simulink model "Pouziti_Discrete"  (R2020b)
settings: Solver=VariableStepAuto  StartTime=0.0  StopTime=10.0  RelTol=1e-3  EnableMultiTasking=on
PreLoadFcn:
  | T = 1;
  | Ts = 0.1;
CloseFcn:
  | clear T Ts
settings Model: Creator=Jirkovsk  LastModifiedBy=jirkovsky
settings DataIOCC: SaveTime=off  ReturnWorkspaceOutputs=off
settings OptimizationCC: LifeSpan=inf
settings DebuggingCC: SFUnexpectedBacktrackingDiag=warning  SFNoUnconditionalDefaultTransitionDiag=warning  SFExecutionAtInitializationDiag=none  ArithmeticOperatorsInVariantConditions=warning
settings SFSimCC: SimUseLocalCustomCode=off  CustomCodeUndefinedFunction=UseInterfaceOnly
settings RTWCC: RTWUseLocalCustomCode=off
settings CodeAppCC: StateflowObjectComments=on
settings GRTTargetCC: TargetLangStandard=C89/C90 (ANSI)
settings ConfigComp: CovMetricSettings=dw  CovSaveCumulativeToWorkspaceVar=on  CovSaveSingleToWorkspaceVar=on  CovExternalEMLEnable=off

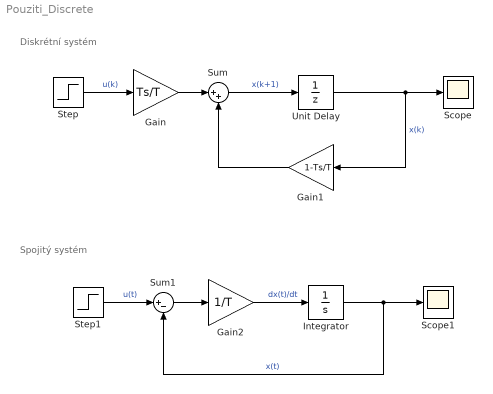
== system Pouziti_Discrete ==
  note: Diskrétní systém
  note: Spojitý systém
  Gain : Gain  Gain=Ts/T
  Gain1 : Gain  Gain=1-Ts/T
  Gain2 : Gain  Gain=1/T
  Integrator : Integrator
  Scope : Scope
  Scope1 : Scope
  Step : Step  SampleTime=Ts
  Step1 : Step  SampleTime=0
  Sum : Sum  Inputs=|++
  Sum1 : Sum  Inputs=|+-
  Unit Delay : UnitDelay  SampleTime=Ts  HasFrameUpgradeWarning=on
  wires:
  Step/1 -> Gain/1  "u(k)"
  Gain/1 -> Sum/1
  Sum/1 -> Unit Delay/1  "x(k+1)"
  Gain1/1 -> Sum/2
  Gain2/1 -> Integrator/1  "dx(t)/dt"
  Sum1/1 -> Gain2/1
  Step1/1 -> Sum1/1  "u(t)"
  Integrator/1 -> Scope1/1, Sum1/2  "x(t)"
  Unit Delay/1 -> Scope/1, Gain1/1  "x(k)"
